simulink model "IntegratedModel"  (R2018b)
settings: Solver=ode1  StartTime=0.0  StopTime=sim.endTime_s  FixedStep=sim.timestep_s  RelTol=1e-3
undefined symbols (not defined in the file): cont, env, sim, vehicle, world
libraries: simulink x9
settings Model: Creator=ogihara  LastModifiedBy=ogihara

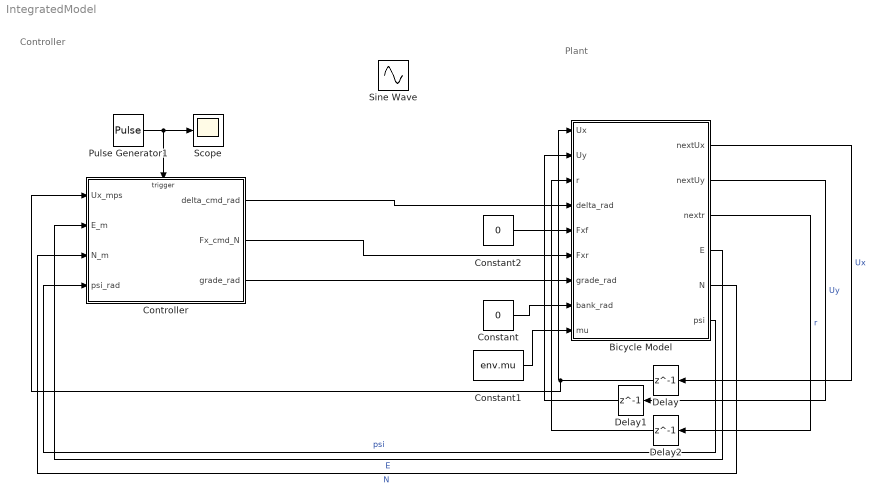
== system IntegratedModel ==
  note: Controller
  note: Plant
  Bicycle Model : Subsystem
  Constant : Constant  Value=0
  Constant1 : Constant  Value=env.mu
  Constant2 : Constant  Value=0
  Controller : Subsystem
  Delay : Delay  DelayLength=1
  Delay1 : Delay  DelayLength=1
  Delay2 : Delay  DelayLength=1
  Pulse Generator1 : DiscretePulseGenerator  PulseType=Time based  Period=cont.period  PulseWidth=10  SampleTime=sim.timestep_s
  Scope : Scope
  Sine Wave : Sin  Amplitude=20/180*pi  Frequency=1.5  SampleTime=0
  wires:
  Bicycle Model/1(nextUx) -> Delay/1  "Ux"
  Bicycle Model/2(nextUy) -> Delay1/1  "Uy"
  Bicycle Model/3(nextr) -> Delay2/1  "r"
  Bicycle Model/4(E) -> Controller/2(E_m)  "E"
  Bicycle Model/5(N) -> Controller/3(N_m)  "N"
  Bicycle Model/6(psi) -> Controller/4(psi_rad)  "psi"
  Constant1/1 -> Bicycle Model/9(mu)
  Constant/1 -> Bicycle Model/8(bank_rad)
  Delay/1 -> Bicycle Model/1(Ux), Controller/1(Ux_mps)
  Delay1/1 -> Bicycle Model/2(Uy)
  Delay2/1 -> Bicycle Model/3(r)
  Controller/3(grade_rad) -> Bicycle Model/7(grade_rad)
  Controller/2(Fx_cmd_N) -> Bicycle Model/6(Fxr)
  Controller/1(delta_cmd_rad) -> Bicycle Model/4(delta_rad)
  Constant2/1 -> Bicycle Model/5(Fxf)
  Pulse Generator1/1 -> Controller/Trigger, Scope/1

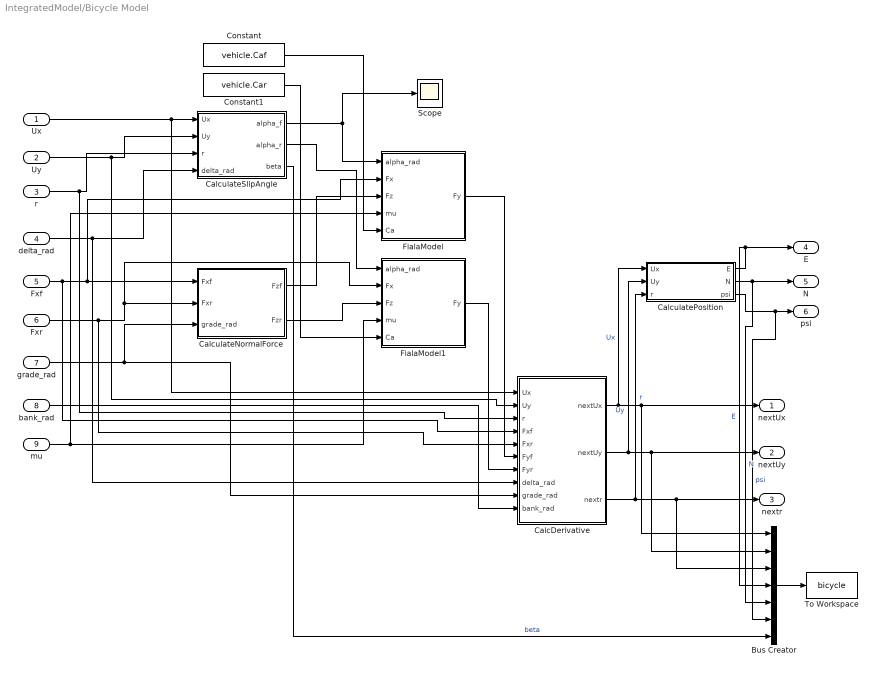
== system IntegratedModel/Bicycle Model ==
  Ux : Inport
  Uy : Inport  Port=2
  r : Inport  Port=3
  delta_rad : Inport  Port=4
  Fxf : Inport  Port=5
  Fxr : Inport  Port=6
  grade_rad : Inport  Port=7
  bank_rad : Inport  Port=8
  mu : Inport  Port=9
  Bus Creator : BusCreator  Inputs=7
  CalcDerivative : Subsystem
  CalculateNormalForce : Subsystem
  CalculatePosition : Subsystem
  CalculateSlipAngle : Subsystem
  Constant : Constant  Value=vehicle.Caf
  Constant1 : Constant  Value=vehicle.Car
  FialaModel : Subsystem
  FialaModel1 : Subsystem
  Scope : Scope
  To Workspace : ToWorkspace  VariableName=bicycle  SaveFormat=Timeseries  SampleTime=-1
  nextUx : Outport
  nextUy : Outport  Port=2
  nextr : Outport  Port=3
  E : Outport  Port=4
  N : Outport  Port=5
  psi : Outport  Port=6
  wires:
  Ux/1 -> CalcDerivative/1(Ux), CalculateSlipAngle/1(Ux)
  Uy/1 -> CalcDerivative/2(Uy), CalculateSlipAngle/2(Uy)
  r/1 -> CalcDerivative/3(r), CalculateSlipAngle/3(r)
  delta_rad/1 -> CalcDerivative/8(delta_rad), CalculateSlipAngle/4(delta_rad)
  Fxf/1 -> FialaModel/2(Fx), CalculateNormalForce/1(Fxf), CalcDerivative/4(Fxf)
  Fxr/1 -> FialaModel1/2(Fx), CalculateNormalForce/2(Fxr), CalcDerivative/5(Fxr)
  grade_rad/1 -> CalcDerivative/9(grade_rad), CalculateNormalForce/3(grade_rad)
  bank_rad/1 -> CalcDerivative/10(bank_rad)
  CalculateSlipAngle/1(alpha_f) -> FialaModel/1(alpha_rad), Scope/1
  CalculateSlipAngle/2(alpha_r) -> FialaModel1/1(alpha_rad)
  CalculateNormalForce/1(Fzf) -> FialaModel/3(Fz)
  mu/1 -> FialaModel1/4(mu), FialaModel/4(mu)
  Constant1/1 -> FialaModel1/5(Ca)
  Constant/1 -> FialaModel/5(Ca)
  CalculateNormalForce/2(Fzr) -> FialaModel1/3(Fz)
  FialaModel/1(Fy) -> CalcDerivative/6(Fyf)
  FialaModel1/1(Fy) -> CalcDerivative/7(Fyr)
  CalculatePosition/1(E) -> E/1, Bus Creator/4  "E"
  CalculatePosition/2(N) -> N/1, Bus Creator/5  "N"
  Bus Creator/1 -> To Workspace/1
  CalcDerivative/3(nextr) -> CalculatePosition/3(r), Bus Creator/3, nextr/1  "r"
  CalcDerivative/1("nextUx ") -> CalculatePosition/1(Ux), nextUx/1, Bus Creator/1  "Ux"
  CalcDerivative/2(nextUy) -> nextUy/1, Bus Creator/2, CalculatePosition/2(Uy)  "Uy"
  CalculatePosition/3(psi) -> Bus Creator/6, psi/1  "psi"
  CalculateSlipAngle/3(beta) -> Bus Creator/7  "beta"

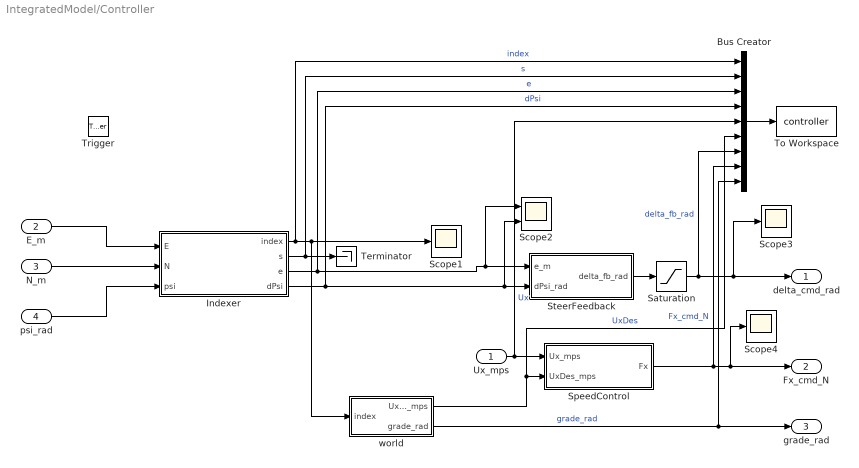
== system IntegratedModel/Controller ==
  Ux_mps : Inport
  E_m : Inport  Port=2
  N_m : Inport  Port=3
  psi_rad : Inport  Port=4
  Trigger : TriggerPort  VariantControl=Variant  PortDimensions=1
  Bus Creator : BusCreator  Inputs=9
  Indexer : Subsystem
  Saturation : Saturate  UpperLimit=vehicle.deltaMax_rad  LowerLimit=-vehicle.deltaMax_rad
  Scope1 : Scope
  Scope2 : Scope  NumInputPorts=2
  Scope3 : Scope
  Scope4 : Scope
  SpeedControl : Subsystem
  SteerFeedback : Subsystem
  Terminator : Terminator
  To Workspace : ToWorkspace  VariableName=controller  SaveFormat=Timeseries  SampleTime=-1
  world : Subsystem
  delta_cmd_rad : Outport
  Fx_cmd_N : Outport  Port=2
  grade_rad : Outport  Port=3
  wires:
  psi_rad/1 -> Indexer/3(psi)
  Indexer/1(index) -> Bus Creator/1, Scope1/1, world/1(index)  "index"
  Indexer/4(dPsi) -> Bus Creator/4, Scope2/2, SteerFeedback/2(dPsi_rad)  "dPsi"
  Indexer/3(e) -> Bus Creator/3, Scope2/1, SteerFeedback/1(e_m)  "e"
  Indexer/2(s) -> Bus Creator/2, Terminator/1  "s"
  SpeedControl/1(Fx) -> Bus Creator/8, Scope4/1, Fx_cmd_N/1  "Fx_cmd_N"
  world/2(grade_rad) -> Bus Creator/9, grade_rad/1  "grade_rad"
  Saturation/1 -> Bus Creator/7, Scope3/1, delta_cmd_rad/1  "delta_fb_rad"
  E_m/1 -> Indexer/1(E)
  N_m/1 -> Indexer/2(N)
  world/1(UxDes_mps) -> Bus Creator/6, SpeedControl/2(UxDes_mps)  "UxDes"
  Ux_mps/1 -> Bus Creator/5, SpeedControl/1(Ux_mps)  "Ux"
  SteerFeedback/1(delta_fb_rad) -> Saturation/1
  Bus Creator/1 -> To Workspace/1

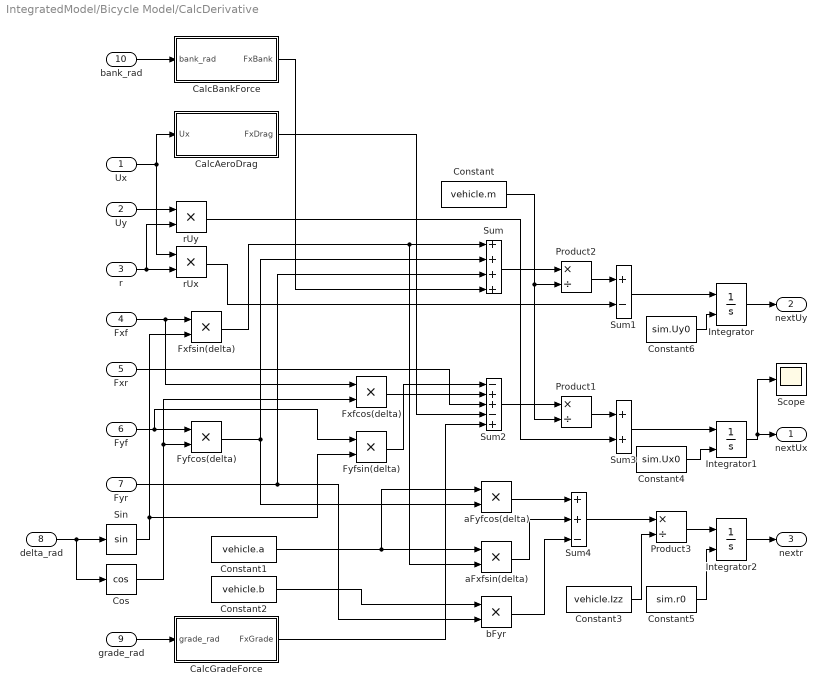
== system IntegratedModel/Bicycle Model/CalcDerivative ==
  Ux : Inport
  Uy : Inport  Port=2
  r : Inport  Port=3
  Fxf : Inport  Port=4
  Fxr : Inport  Port=5
  Fyf : Inport  Port=6
  Fyr : Inport  Port=7
  delta_rad : Inport  Port=8
  grade_rad : Inport  Port=9
  bank_rad : Inport  Port=10
  CalcAeroDrag : Subsystem
  CalcBankForce : Subsystem
  CalcGradeForce : Subsystem
  Constant : Constant  Value=vehicle.m
  Constant1 : Constant  Value=vehicle.a
  Constant2 : Constant  Value=vehicle.b
  Constant3 : Constant  Value=vehicle.Izz
  Constant4 : Constant  Value=sim.Ux0
  Constant5 : Constant  Value=sim.r0
  Constant6 : Constant  Value=sim.Uy0
  Cos : Trigonometry  Operator=cos
  Fxfcos(delta) : Product
  Fxfsin(delta) : Product
  Fyfcos(delta) : Product
  Fyfsin(delta) : Product
  Integrator : Integrator  InitialConditionSource=external
  Integrator1 : Integrator  InitialConditionSource=external
  Integrator2 : Integrator  InitialConditionSource=external  InitialCondition=sim.r0
  Product1 : Product  Inputs=*/
  Product2 : Product  Inputs=*/
  Product3 : Product  Inputs=*/
  Scope : Scope
  Sin : Trigonometry
  Sum : Sum  Inputs=++++
  Sum1 : Sum  Inputs=+-
  Sum2 : Sum  Inputs=-++-+
  Sum3 : Sum
  Sum4 : Sum  Inputs=++-
  aFxfsin(delta) : Product
  aFyfcos(delta) : Product
  bFyr : Product
  rUx : Product
  rUy : Product
  "nextUx " : Outport
  nextUy : Outport  Port=2
  nextr : Outport  Port=3
  wires:
  delta_rad/1 -> Cos/1, Sin/1
  Fyf/1 -> Fyfsin(delta)/1, Fyfcos(delta)/1
  Cos/1 -> Fxfcos(delta)/2, Fyfcos(delta)/2
  Fxf/1 -> Fxfcos(delta)/1, Fxfsin(delta)/1
  Sin/1 -> Fyfsin(delta)/2, Fxfsin(delta)/2
  Fxfsin(delta)/1 -> Sum/1, aFxfsin(delta)/2
  Fyfcos(delta)/1 -> aFyfcos(delta)/2, Sum/2
  Fyr/1 -> bFyr/2, Sum/3
  grade_rad/1 -> CalcGradeForce/1(grade_rad)
  Constant/1 -> Product1/2, Product2/2
  Sum/1 -> Product2/1
  r/1 -> rUx/2, rUy/2
  Ux/1 -> CalcAeroDrag/1(Ux), rUx/1
  Product2/1 -> Sum1/1
  Sum1/1 -> Integrator/1
  rUx/1 -> Sum1/2
  Uy/1 -> rUy/1
  bank_rad/1 -> CalcBankForce/1(bank_rad)
  CalcBankForce/1(FxBank) -> Sum/4
  Fxr/1 -> Sum2/3
  CalcAeroDrag/1(FxDrag) -> Sum2/4
  CalcGradeForce/1(FxGrade) -> Sum2/5
  Sum3/1 -> Integrator1/1
  Product1/1 -> Sum3/1
  Sum2/1 -> Product1/1
  rUy/1 -> Sum3/2
  Constant1/1 -> aFxfsin(delta)/1, aFyfcos(delta)/1
  Constant2/1 -> bFyr/1
  aFyfcos(delta)/1 -> Sum4/1
  aFxfsin(delta)/1 -> Sum4/2
  bFyr/1 -> Sum4/3
  Constant3/1 -> Product3/2
  Sum4/1 -> Product3/1
  Product3/1 -> Integrator2/1
  Integrator/1 -> nextUy/1
  Integrator1/1 -> Scope/1, "nextUx "/1
  Integrator2/1 -> nextr/1
  Constant4/1 -> Integrator1/2
  Constant5/1 -> Integrator2/2
  Constant6/1 -> Integrator/2
  Fyfsin(delta)/1 -> Sum2/1
  Fxfcos(delta)/1 -> Sum2/2

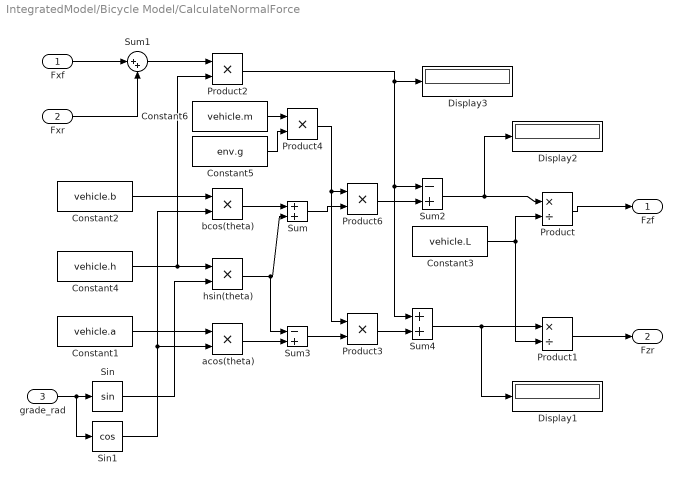
== system IntegratedModel/Bicycle Model/CalculateNormalForce ==
  Fxf : Inport
  Fxr : Inport  Port=2
  grade_rad : Inport  Port=3
  Constant1 : Constant  Value=vehicle.a
  Constant2 : Constant  Value=vehicle.b
  Constant3 : Constant  Value=vehicle.L
  Constant4 : Constant  Value=vehicle.h
  Constant5 : Constant  Value=env.g
  Constant6 : Constant  Value=vehicle.m
  Display1 : Display
  Display2 : Display
  Display3 : Display
  Product : Product  Inputs=*/
  Product1 : Product  Inputs=*/
  Product{2..4,6} (4 alike) : Product
  Sin : Trigonometry
  Sin1 : Trigonometry  Operator=cos
  Sum : Sum
  Sum1 : Sum  Inputs=|++
  Sum2 : Sum  Inputs=-+
  Sum3 : Sum  Inputs=-+
  Sum4 : Sum
  acos(theta) : Product
  bcos(theta) : Product
  hsin(theta) : Product
  Fzf : Outport
  Fzr : Outport  Port=2
  wires:
  grade_rad/1 -> Sin1/1, Sin/1
  Constant2/1 -> bcos(theta)/1
  Sin1/1 -> bcos(theta)/2, acos(theta)/2
  Constant1/1 -> acos(theta)/1
  Sin/1 -> hsin(theta)/2
  bcos(theta)/1 -> Sum/1
  hsin(theta)/1 -> Sum3/1, Sum/2
  Sum/1 -> Product6/2
  Fxf/1 -> Sum1/1
  Fxr/1 -> Sum1/2
  Constant4/1 -> Product2/2, hsin(theta)/1
  Sum1/1 -> Product2/1
  Product6/1 -> Sum2/2
  Product2/1 -> Display3/1, Sum4/1, Sum2/1
  Sum2/1 -> Display2/1, Product/1
  Product/1 -> Fzf/1
  acos(theta)/1 -> Sum3/2
  Sum4/1 -> Display1/1, Product1/1
  Product3/1 -> Sum4/2
  Sum3/1 -> Product3/2
  Product1/1 -> Fzr/1
  Constant6/1 -> Product4/1
  Constant5/1 -> Product4/2
  Product4/1 -> Product3/1, Product6/1
  Constant3/1 -> Product1/2, Product/2

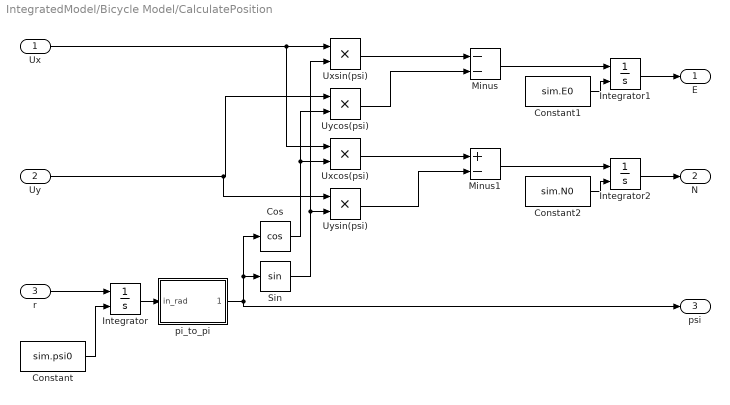
== system IntegratedModel/Bicycle Model/CalculatePosition ==
  Ux : Inport
  Uy : Inport  Port=2
  r : Inport  Port=3
  Constant : Constant  Value=sim.psi0
  Constant1 : Constant  Value=sim.E0
  Constant2 : Constant  Value=sim.N0
  Cos : Trigonometry  Operator=cos
  Integrator : Integrator  InitialConditionSource=external
  Integrator1 : Integrator  InitialConditionSource=external
  Integrator2 : Integrator  InitialConditionSource=external
  Minus : Sum  Inputs=--
  Minus1 : Sum  Inputs=+-
  Sin : Trigonometry
  Uxcos(psi) : Product
  Uxsin(psi) : Product
  Uycos(psi) : Product
  Uysin(psi) : Product
  pi_to_pi : Subsystem
  E : Outport
  N : Outport  Port=2
  psi : Outport  Port=3
  wires:
  r/1 -> Integrator/1
  Constant/1 -> Integrator/2
  Integrator/1 -> pi_to_pi/1(in_rad)
  Integrator1/1 -> E/1
  Constant1/1 -> Integrator1/2
  Ux/1 -> Uxcos(psi)/1, Uxsin(psi)/1
  Sin/1 -> Uysin(psi)/2, Uxsin(psi)/2
  Uy/1 -> Uysin(psi)/1, Uycos(psi)/1
  Cos/1 -> Uxcos(psi)/2, Uycos(psi)/2
  Uxsin(psi)/1 -> Minus/1
  Uycos(psi)/1 -> Minus/2
  Minus/1 -> Integrator1/1
  Uxcos(psi)/1 -> Minus1/1
  Uysin(psi)/1 -> Minus1/2
  Minus1/1 -> Integrator2/1
  Constant2/1 -> Integrator2/2
  Integrator2/1 -> N/1
  pi_to_pi/1(out_rad) -> Sin/1, Cos/1, psi/1

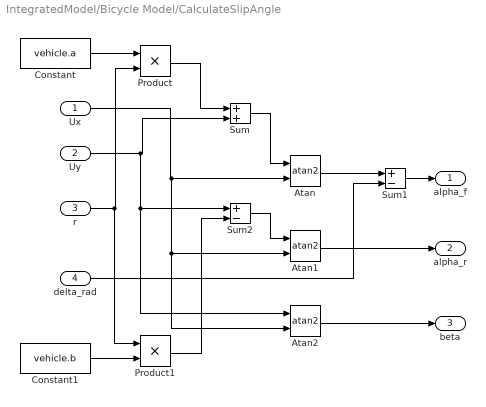
== system IntegratedModel/Bicycle Model/CalculateSlipAngle ==
  Ux : Inport
  Uy : Inport  Port=2
  r : Inport  Port=3
  delta_rad : Inport  Port=4
  Atan : Trigonometry  Operator=atan2
  Atan1 : Trigonometry  Operator=atan2
  Atan2 : Trigonometry  Operator=atan2
  Constant : Constant  Value=vehicle.a
  Constant1 : Constant  Value=vehicle.b
  Product : Product
  Product1 : Product
  Sum : Sum
  Sum1 : Sum  Inputs=+-
  Sum2 : Sum  Inputs=+-
  alpha_f : Outport
  alpha_r : Outport  Port=2
  beta : Outport  Port=3
  wires:
  Constant/1 -> Product/1
  r/1 -> Product1/1, Product/2
  Constant1/1 -> Product1/2
  Ux/1 -> Atan2/2, Atan1/2, Atan/2
  Uy/1 -> Atan2/1, Sum2/1, Sum/2
  Product/1 -> Sum/1
  Sum/1 -> Atan/1
  delta_rad/1 -> Sum1/2
  Atan/1 -> Sum1/1
  Sum1/1 -> alpha_f/1
  Product1/1 -> Sum2/2
  Sum2/1 -> Atan1/1
  Atan1/1 -> alpha_r/1
  Atan2/1 -> beta/1

== system IntegratedModel/Bicycle Model/FialaModel ==
  alpha_rad : Inport
  Fx : Inport  Port=2
  Fz : Inport  Port=3
  mu : Inport  Port=4
  Ca : Inport  Port=5
  Bus Creator : BusCreator  Inputs=7
  Switch : Switch  Criteria=u2 > Threshold
  To Workspace : ToWorkspace  VariableName=frontTire  SaveFormat=Timeseries  SampleTime=-1
  isSaturated : Subsystem
  not saturated : Subsystem
  saturated : Subsystem
  Fy : Outport
  wires:
  Switch/1 -> Bus Creator/7, Fy/1  "Fy"
  alpha_rad/1 -> Bus Creator/1, not saturated/1(alpha), isSaturated/1(alpha), saturated/4(alpha)  "alpha"
  Fx/1 -> Bus Creator/2, isSaturated/2(Fx)  "Fx"
  Fz/1 -> Bus Creator/3, not saturated/2(Fz), saturated/3(Fz), isSaturated/3(Fz)  "Fz"
  mu/1 -> saturated/1(mu), not saturated/3(mu), Bus Creator/4, isSaturated/4(mu)  "mu"
  Ca/1 -> not saturated/4(Ca), Bus Creator/5, isSaturated/5(Ca)  "Ca"
  isSaturated/1(saturatedFlag) -> Bus Creator/6, Switch/2  "isSaturated"
  saturated/1(Fy) -> Switch/1
  not saturated/1(Fy) -> Switch/3
  isSaturated/2(zeta) -> saturated/2(zeta), not saturated/5(zeta)
  Bus Creator/1 -> To Workspace/1

== system IntegratedModel/Bicycle Model/FialaModel1 ==
  alpha_rad : Inport
  Fx : Inport  Port=2
  Fz : Inport  Port=3
  mu : Inport  Port=4
  Ca : Inport  Port=5
  Bus Creator : BusCreator  Inputs=7
  Switch : Switch  Criteria=u2 > Threshold
  To Workspace : ToWorkspace  VariableName=rearTire  SaveFormat=Timeseries  SampleTime=-1
  isSaturated : Subsystem
  not saturated : Subsystem
  saturated : Subsystem
  Fy : Outport
  wires:
  Switch/1 -> Bus Creator/7, Fy/1  "Fy"
  alpha_rad/1 -> Bus Creator/1, not saturated/1(alpha), isSaturated/1(alpha), saturated/4(alpha)  "alpha"
  Fx/1 -> Bus Creator/2, isSaturated/2(Fx)  "Fx"
  Fz/1 -> Bus Creator/3, not saturated/2(Fz), saturated/3(Fz), isSaturated/3(Fz)  "Fz"
  mu/1 -> saturated/1(mu), not saturated/3(mu), Bus Creator/4, isSaturated/4(mu)  "mu"
  Ca/1 -> not saturated/4(Ca), Bus Creator/5, isSaturated/5(Ca)  "Ca"
  isSaturated/1(saturatedFlag) -> Bus Creator/6, Switch/2  "isSaturated"
  saturated/1(Fy) -> Switch/1
  not saturated/1(Fy) -> Switch/3
  isSaturated/2(zeta) -> saturated/2(zeta), not saturated/5(zeta)
  Bus Creator/1 -> To Workspace/1

== system IntegratedModel/Controller/Indexer ==
  E : Inport
  N : Inport  Port=2
  psi : Inport  Port=3
  CalcLocalCoordinate : Subsystem
  Delay1 : Delay  DelayLength=1
  FindNearestIndex : Subsystem
  IC1 : InitialCondition
  index : Outport
  s : Outport  Port=2
  e : Outport  Port=3
  dPsi : Outport  Port=4
  wires:
  IC1/1 -> FindNearestIndex/1(currentIndex)
  CalcLocalCoordinate/3(dpsi) -> dPsi/1  "dPsi"
  FindNearestIndex/1(nearestIndex) -> index/1, CalcLocalCoordinate/1(currentIdx), Delay1/1  "index"
  psi/1 -> CalcLocalCoordinate/4(psi)  "psi"
  E/1 -> CalcLocalCoordinate/2(E), FindNearestIndex/2(E)  "E"
  Delay1/1 -> IC1/1
  CalcLocalCoordinate/1(s) -> s/1  "s"
  N/1 -> CalcLocalCoordinate/3(N), FindNearestIndex/3(N)  "N"
  CalcLocalCoordinate/2(e) -> e/1  "e"

== system IntegratedModel/Controller/SpeedControl ==
  Ux_mps : Inport
  UxDes_mps : Inport  Port=2
  Gain : Gain  Gain=cont.accel_gain
  SpeedFeedback : Subsystem
  Fx : Outport
  wires:
  Ux_mps/1 -> SpeedFeedback/1(Ux_mps)
  UxDes_mps/1 -> SpeedFeedback/2(UxDes_mps)
  SpeedFeedback/1(LonCmd (-1,1)) -> Gain/1
  Gain/1 -> Fx/1  "Fx"

== system IntegratedModel/Controller/SteerFeedback ==
  e_m : Inport
  dPsi_rad : Inport  Port=2
  Gain : Gain  Gain=cont.x_la
  Gain1 : Gain  Gain=cont.k_fb
  Plus : Sum
  delta_fb_rad : Outport
  wires:
  dPsi_rad/1 -> Gain/1
  e_m/1 -> Plus/1
  Gain/1 -> Plus/2
  Plus/1 -> Gain1/1
  Gain1/1 -> delta_fb_rad/1

== system IntegratedModel/Controller/world ==
  index : Inport
  world.UxDes_mps : Lookup_n-D  NumberOfTableDimensions=1  BreakpointsForDimension1=world.index  Table=world.UxDes_mps  InternalRulePriority=Speed  RndMeth=Simplest  InputSameDT=on
  world.grade_rad : Lookup_n-D  NumberOfTableDimensions=1  BreakpointsForDimension1=world.index  Table=world.grade_rad  InternalRulePriority=Speed  RndMeth=Simplest  InputSameDT=on
  UxDes_mps : Outport
  grade_rad : Outport  Port=2
  wires:
  index/1 -> world.UxDes_mps/1, world.grade_rad/1
  world.grade_rad/1 -> grade_rad/1  "grade"
  world.UxDes_mps/1 -> UxDes_mps/1  "UxDes"

== system IntegratedModel/Bicycle Model/CalcDerivative/CalcAeroDrag ==
  Ux : Inport
  Constant : Constant  Value=vehicle.Cd0
  Gain : Gain  Gain=vehicle.Cd1
  Gain1 : Gain  Gain=vehicle.Cd2
  Product : Product
  Product1 : Product
  Sign : Signum
  Square : Math  Operator=square  SaturateOnIntegerOverflow=on
  Sum : Sum  Inputs=3
  FxDrag : Outport
  wires:
  Sum/1 -> FxDrag/1
  Gain1/1 -> Product1/2
  Gain/1 -> Sum/2
  Square/1 -> Gain1/1
  Ux/1 -> Gain/1, Square/1, Sign/1
  Product/1 -> Sum/1
  Sign/1 -> Product1/1, Product/2
  Constant/1 -> Product/1
  Product1/1 -> Sum/3

== system IntegratedModel/Bicycle Model/CalcDerivative/CalcBankForce ==
  bank_rad : Inport
  Constant : Constant  Value=vehicle.m
  Constant1 : Constant  Value=env.g
  Product : Product  Inputs=3
  Sin : Trigonometry
  FxBank : Outport
  wires:
  bank_rad/1 -> Sin/1
  Sin/1 -> Product/1
  Constant/1 -> Product/2
  Constant1/1 -> Product/3
  Product/1 -> FxBank/1

== system IntegratedModel/Bicycle Model/CalcDerivative/CalcGradeForce ==
  grade_rad : Inport
  Constant : Constant  Value=vehicle.m
  Constant1 : Constant  Value=env.g
  Product : Product  Inputs=3
  Sin : Trigonometry
  FxGrade : Outport
  wires:
  grade_rad/1 -> Sin/1
  Sin/1 -> Product/1
  Constant/1 -> Product/2
  Constant1/1 -> Product/3
  Product/1 -> FxGrade/1

== system IntegratedModel/Bicycle Model/CalculatePosition/pi_to_pi ==
  in_rad : Inport
  Compare To Constant : simulink/Logic and Bit Operations/Compare To Constant  relop=<=  const=-pi  OutDataTypeStr=boolean
  Compare To Constant1 : simulink/Logic and Bit Operations/Compare To Constant  relop=>  const=pi  OutDataTypeStr=boolean
  Constant : Constant  Value=2*pi
  Minus : Sum  Inputs=+-
  Plus : Sum
  Switch : Switch  Criteria=u2 > Threshold
  Switch1 : Switch  Criteria=u2 > Threshold
  out_rad : Outport
  wires:
  Constant/1 -> Minus/2, Plus/2
  in_rad/1 -> Switch/3, Compare To Constant/1, Minus/1, Plus/1
  Compare To Constant1/1 -> Switch1/2
  Compare To Constant/1 -> Switch/2
  Plus/1 -> Switch/1
  Switch/1 -> Switch1/3, Compare To Constant1/1
  Minus/1 -> Switch1/1
  Switch1/1 -> out_rad/1

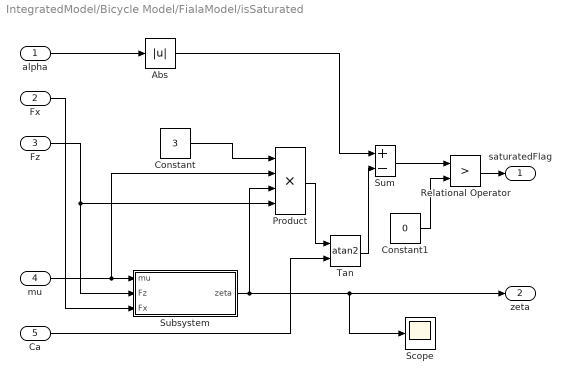
== system IntegratedModel/Bicycle Model/FialaModel/isSaturated ==
  alpha : Inport
  Fx : Inport  Port=2
  Fz : Inport  Port=3
  mu : Inport  Port=4
  Ca : Inport  Port=5
  Abs : Abs
  Constant : Constant  Value=3
  Constant1 : Constant  Value=0
  Product : Product  Inputs=4
  Relational Operator : RelationalOperator  Operator=>  OutDataTypeStr=boolean  RndMeth=Simplest
  Scope : Scope
  Subsystem : Subsystem
  Sum : Sum  Inputs=+-
  Tan : Trigonometry  Operator=atan2
  saturatedFlag : Outport
  zeta : Outport  Port=2
  wires:
  Subsystem/1(zeta) -> Scope/1, zeta/1, Product/3
  Product/1 -> Tan/1
  Tan/1 -> Sum/2
  Fx/1 -> Subsystem/3(Fx)
  Fz/1 -> Subsystem/2(Fz), Product/4
  Constant/1 -> Product/1
  mu/1 -> Product/2, Subsystem/1(mu)
  Ca/1 -> Tan/2
  Abs/1 -> Sum/1
  alpha/1 -> Abs/1
  Sum/1 -> Relational Operator/1
  Constant1/1 -> Relational Operator/2
  Relational Operator/1 -> saturatedFlag/1

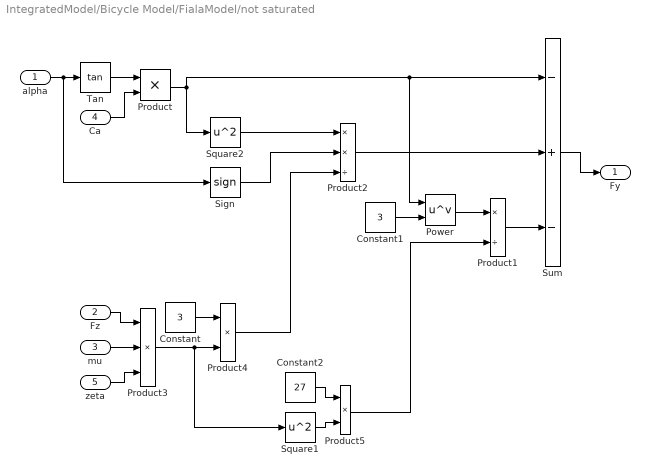
== system IntegratedModel/Bicycle Model/FialaModel/not saturated ==
  alpha : Inport
  Fz : Inport  Port=2
  mu : Inport  Port=3
  Ca : Inport  Port=4
  zeta : Inport  Port=5
  Constant : Constant  Value=3
  Constant1 : Constant  Value=3
  Constant2 : Constant  Value=27
  Power : Math  Operator=pow  SaturateOnIntegerOverflow=on
  Product : Product
  Product1 : Product  Inputs=*/
  Product2 : Product  Inputs=**/
  Product3 : Product  Inputs=***
  Product4 : Product
  Product5 : Product
  Sign : Signum
  Square1 : Math  Operator=square  SaturateOnIntegerOverflow=on
  Square2 : Math  Operator=square  SaturateOnIntegerOverflow=on
  Sum : Sum  Inputs=-+-
  Tan : Trigonometry  Operator=tan
  Fy : Outport
  wires:
  Sum/1 -> Fy/1
  alpha/1 -> Sign/1, Tan/1
  Tan/1 -> Product/1
  Ca/1 -> Product/2
  Product/1 -> Square2/1, Power/1, Sum/1
  Square2/1 -> Product2/1
  Product2/1 -> Sum/2
  Fz/1 -> Product3/1
  mu/1 -> Product3/2
  zeta/1 -> Product3/3
  Product3/1 -> Square1/1, Product4/2
  Constant/1 -> Product4/1
  Product4/1 -> Product2/3
  Sign/1 -> Product2/2
  Constant2/1 -> Product5/1
  Square1/1 -> Product5/2
  Constant1/1 -> Power/2
  Power/1 -> Product1/1
  Product5/1 -> Product1/2
  Product1/1 -> Sum/3

== system IntegratedModel/Bicycle Model/FialaModel/saturated ==
  mu : Inport
  zeta : Inport  Port=2
  Fz : Inport  Port=3
  alpha : Inport  Port=4
  Gain : Gain  Gain=-1
  Product : Product  Inputs=4
  Sign : Signum
  Fy : Outport
  wires:
  alpha/1 -> Sign/1
  Product/1 -> Gain/1
  Gain/1 -> Fy/1
  mu/1 -> Product/1
  zeta/1 -> Product/2
  Fz/1 -> Product/3
  Sign/1 -> Product/4

== system IntegratedModel/Bicycle Model/FialaModel1/isSaturated ==
  alpha : Inport
  Fx : Inport  Port=2
  Fz : Inport  Port=3
  mu : Inport  Port=4
  Ca : Inport  Port=5
  Abs : Abs
  Constant : Constant  Value=3
  Constant1 : Constant  Value=0
  Product : Product  Inputs=4
  Relational Operator : RelationalOperator  Operator=>  OutDataTypeStr=boolean  RndMeth=Simplest
  Scope : Scope
  Subsystem : Subsystem
  Sum : Sum  Inputs=+-
  Tan : Trigonometry  Operator=atan2
  saturatedFlag : Outport
  zeta : Outport  Port=2
  wires:
  Subsystem/1(zeta) -> Scope/1, zeta/1, Product/3
  Product/1 -> Tan/1
  Tan/1 -> Sum/2
  Fx/1 -> Subsystem/3(Fx)
  Fz/1 -> Subsystem/2(Fz), Product/4
  Constant/1 -> Product/1
  mu/1 -> Product/2, Subsystem/1(mu)
  Ca/1 -> Tan/2
  Abs/1 -> Sum/1
  alpha/1 -> Abs/1
  Sum/1 -> Relational Operator/1
  Constant1/1 -> Relational Operator/2
  Relational Operator/1 -> saturatedFlag/1

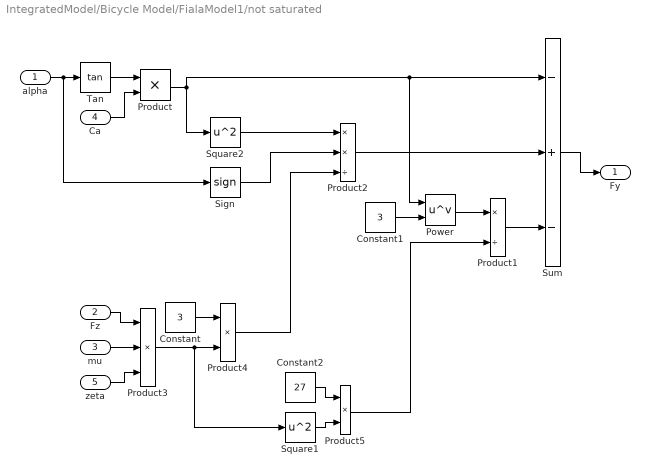
== system IntegratedModel/Bicycle Model/FialaModel1/not saturated ==
  alpha : Inport
  Fz : Inport  Port=2
  mu : Inport  Port=3
  Ca : Inport  Port=4
  zeta : Inport  Port=5
  Constant : Constant  Value=3
  Constant1 : Constant  Value=3
  Constant2 : Constant  Value=27
  Power : Math  Operator=pow  SaturateOnIntegerOverflow=on
  Product : Product
  Product1 : Product  Inputs=*/
  Product2 : Product  Inputs=**/
  Product3 : Product  Inputs=***
  Product4 : Product
  Product5 : Product
  Sign : Signum
  Square1 : Math  Operator=square  SaturateOnIntegerOverflow=on
  Square2 : Math  Operator=square  SaturateOnIntegerOverflow=on
  Sum : Sum  Inputs=-+-
  Tan : Trigonometry  Operator=tan
  Fy : Outport
  wires:
  Sum/1 -> Fy/1
  alpha/1 -> Sign/1, Tan/1
  Tan/1 -> Product/1
  Ca/1 -> Product/2
  Product/1 -> Square2/1, Power/1, Sum/1
  Square2/1 -> Product2/1
  Product2/1 -> Sum/2
  Fz/1 -> Product3/1
  mu/1 -> Product3/2
  zeta/1 -> Product3/3
  Product3/1 -> Square1/1, Product4/2
  Constant/1 -> Product4/1
  Product4/1 -> Product2/3
  Sign/1 -> Product2/2
  Constant2/1 -> Product5/1
  Square1/1 -> Product5/2
  Constant1/1 -> Power/2
  Power/1 -> Product1/1
  Product5/1 -> Product1/2
  Product1/1 -> Sum/3

== system IntegratedModel/Bicycle Model/FialaModel1/saturated ==
  mu : Inport
  zeta : Inport  Port=2
  Fz : Inport  Port=3
  alpha : Inport  Port=4
  Gain : Gain  Gain=-1
  Product : Product  Inputs=4
  Sign : Signum
  Fy : Outport
  wires:
  alpha/1 -> Sign/1
  Product/1 -> Gain/1
  Gain/1 -> Fy/1
  mu/1 -> Product/1
  zeta/1 -> Product/2
  Fz/1 -> Product/3
  Sign/1 -> Product/4

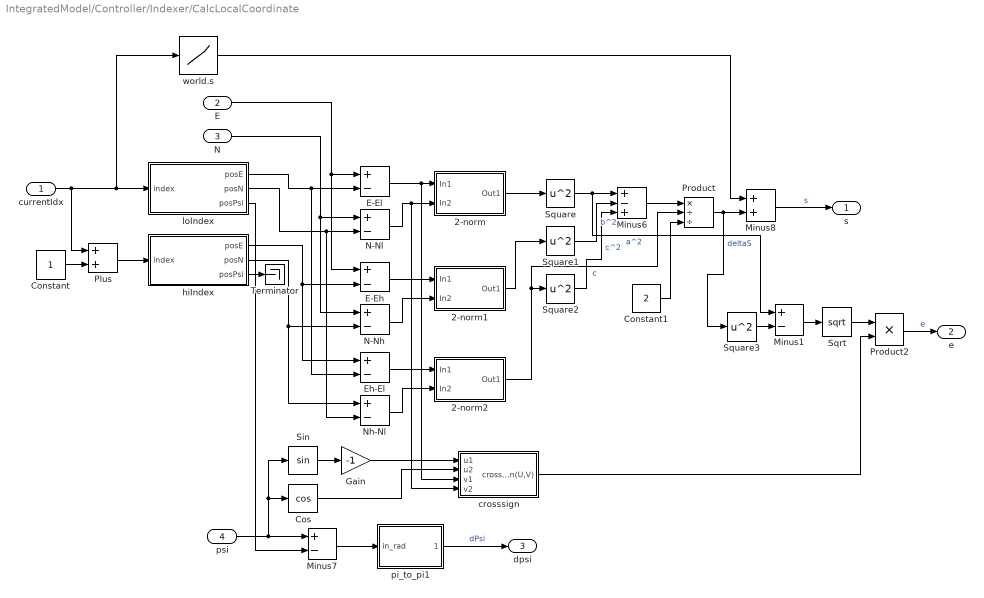
== system IntegratedModel/Controller/Indexer/CalcLocalCoordinate ==
  currentIdx : Inport
  E : Inport  Port=2
  N : Inport  Port=3
  psi : Inport  Port=4
  2-norm : Subsystem
  2-norm1 : Subsystem
  2-norm2 : Subsystem
  Constant : Constant
  Constant1 : Constant  Value=2
  Cos : Trigonometry  Operator=cos
  E-Eh : Sum  Inputs=+-
  E-El : Sum  Inputs=+-
  Eh-El : Sum  Inputs=+-
  Gain : Gain  Gain=-1
  Minus1 : Sum  Inputs=+-
  Minus6 : Sum  Inputs=+-+
  Minus7 : Sum  Inputs=+-
  Minus8 : Sum
  N-Nh : Sum  Inputs=+-
  N-Nl : Sum  Inputs=+-
  Nh-Nl : Sum  Inputs=+-
  Plus : Sum
  Product : Product  Inputs=*//
  Product2 : Product
  Sin : Trigonometry
  Sqrt : Sqrt  SaturateOnIntegerOverflow=on
  Square{,1..3} (4 alike) : Math  Operator=square  SaturateOnIntegerOverflow=on
  Terminator : Terminator
  crosssign : Subsystem
  hiIndex : Subsystem
  loIndex : Subsystem
  pi_to_pi1 : Subsystem
  world.s : Lookup_n-D  NumberOfTableDimensions=1  BreakpointsForDimension1=world.index  Table=world.s_m  InternalRulePriority=Speed  RndMeth=Simplest  InputSameDT=on
  s : Outport
  e : Outport  Port=2
  dpsi : Outport  Port=3
  wires:
  currentIdx/1 -> Plus/1, world.s/1, loIndex/1(index)
  Constant/1 -> Plus/2
  Plus/1 -> hiIndex/1(index)
  hiIndex/3(posPsi) -> Terminator/1
  hiIndex/1(posE) -> Eh-El/1, E-Eh/2
  E-El/1 -> crosssign/3(v1), 2-norm/1(In1)
  N-Nl/1 -> crosssign/4(v2), 2-norm/2(In2)
  E-Eh/1 -> 2-norm1/1(In1)
  N-Nh/1 -> 2-norm1/2(In2)
  Eh-El/1 -> 2-norm2/1(In1)
  Nh-Nl/1 -> 2-norm2/2(In2)
  2-norm/1(Out1) -> Square/1
  2-norm1/1(Out1) -> Square1/1
  2-norm2/1(Out1) -> Product/2, Square2/1  "c"
  Square/1 -> Minus1/1, Minus6/1  "a^2"
  Square1/1 -> Minus6/2  "b^2"
  Square2/1 -> Minus6/3  "c^2"
  Minus6/1 -> Product/1
  Constant1/1 -> Product/3
  psi/1 -> Cos/1, Sin/1, Minus7/1
  Minus7/1 -> pi_to_pi1/1(in_rad)
  Product/1 -> Square3/1, Minus8/2  "deltaS"
  world.s/1 -> Minus8/1
  Minus8/1 -> s/1  "s"
  Sin/1 -> Gain/1
  Gain/1 -> crosssign/1(u1)
  Cos/1 -> crosssign/2(u2)
  E/1 -> E-Eh/1, E-El/1
  loIndex/1(posE) -> Eh-El/2, E-El/2
  loIndex/2(posN) -> Nh-Nl/2, N-Nl/2
  N/1 -> N-Nh/1, N-Nl/1
  hiIndex/2(posN) -> Nh-Nl/1, N-Nh/2
  loIndex/3(posPsi) -> Minus7/2
  Square3/1 -> Minus1/2
  Minus1/1 -> Sqrt/1
  Sqrt/1 -> Product2/1
  Product2/1 -> e/1  "e"
  crosssign/1(crosssign(U,V)) -> Product2/2
  pi_to_pi1/1(out_rad) -> dpsi/1  "dPsi"

== system IntegratedModel/Controller/Indexer/FindNearestIndex ==
  note: Osprey had forward & backward search.
      | This simulator has only forward search and max width is 5.
  currentIndex : Inport
  E : Inport  Port=2
  N : Inport  Port=3
  ForwardSearch : Subsystem  TreatAsAtomicUnit=on
  nearestIndex : Outport
  wires:
  currentIndex/1 -> ForwardSearch/1(CurrentIndex)
  E/1 -> ForwardSearch/2(E)
  N/1 -> ForwardSearch/3(N)
  ForwardSearch/1(loIndexF) -> nearestIndex/1

== system IntegratedModel/Controller/SpeedControl/SpeedFeedback ==
  Ux_mps : Inport
  UxDes_mps : Inport  Port=2
  Gain : Gain  Gain=cont.speed_gain
  PID Controller : simulink/Continuous/PID Controller  Controller=PID  Form=Parallel  TimeDomain=Discrete-time  SampleTime=-1  IntegratorMethod=Forward Euler  FilterMethod=Forward Euler  ControllerParametersSource=internal  P=cont.k_p_speed  I=cont.k_i_speed  D=cont.k_d_speed  UseFilter=on  N=100  TunerSelectOption=Transfer Function Based (PID Tuner App)  InitialConditionSource=internal  InitialConditionForIntegrator=0  InitialConditionForFilter=0  DifferentiatorICPrevScaledInput=0  ExternalReset=none  TrackingMode=off  Kt=1  LimitOutput=off  UpperSaturationLimit=inf  LowerSaturationLimit=-inf  LinearizeAsGain=on  AntiWindupMode=none  Kb=1  POutMin=[]  POutMax=[]  IOutMin=[]  IOutMax=[]  DOutMin=[]  DOutMax=[]  NOutMin=[]  NOutMax=[]  SumOutMin=[]  SumOutMax=[]  SaturationOutMin=[]  SaturationOutMax=[]  PParamMin=[]  PParamMax=[]  IParamMin=[]  IParamMax=[]  DParamMin=[]  DParamMax=[]  NParamMin=[]  NParamMax=[]  KbParamMin=[]  KbParamMax=[]  KtParamMin=[]  KtParamMax=[]  KbOutMin=[]  KbOutMax=[]  KtOutMin=[]  KtOutMax=[]  IntegratorOutMin=[]  IntegratorOutMax=[]  FilterOutMin=[]  FilterOutMax=[]  SumI1OutMin=[]  SumI1OutMax=[]  SumI2OutMin=[]  SumI2OutMax=[]  SumI3OutMin=[]  SumI3OutMax=[]  SumI4OutMin=[]  SumI4OutMax=[]  SumDOutMin=[]  SumDOutMax=[]  DifferentiatorOutMin=[]  DifferentiatorOutMax=[]  FilterDiffOutCoefMin=[]  FilterDiffOutCoefMax=[]  ReciprocalOutMin=[]  ReciprocalOutMax=[]  SumDenOutMin=[]  SumDenOutMax=[]  SumNumOutMin=[]  SumNumOutMax=[]  DivideOutMin=[]  DivideOutMax=[]  IntegratorContinuousStateAttributes=''  IntegratorStateMustResolveToSignalObject=off  IntegratorRTWStateStorageClass=Auto  FilterContinuousStateAttributes=''  FilterStateMustResolveToSignalObject=off  FilterRTWStateStorageClass=Auto  ParallelPVariant=InternalParameters  IdealPVariant=Disabled  IVariant=InternalParameters  DVariant=InternalParameters  IntegratorVariant=Discrete  SatVariant=Disabled  AWVariant=Passthrough  PCopyVariant=Disabled  TRVariant=Disabled  FdbkBlocksVariant=Forward  IdealPFdbkVariant=Disabled  SatFdbkVariant=Disabled  DerivativeFilterVariant=ForwardEulerFilter  NVariant=InternalParameters  NCopyVariant=Disabled  FilterICVariant=InternalICsFilter  IntegratorICVariant=InternalICs  ExternalResetVariant=Disabled  TRSumVariant=Passthrough  SumFdbkVariant=Disabled  SumVariant=Sum_PID
  Plus : Sum  Inputs=+-
  Saturation : Saturate  UpperLimit=+1  LowerLimit=-1
  Scope : Scope  NumInputPorts=2
  LonCmd (-1,1) : Outport
  wires:
  PID Controller/1 -> Gain/1
  Gain/1 -> Saturation/1
  Saturation/1 -> Scope/2, LonCmd (-1,1)/1
  Ux_mps/1 -> Plus/2
  UxDes_mps/1 -> Plus/1
  Plus/1 -> Scope/1, PID Controller/1

== system IntegratedModel/Bicycle Model/FialaModel/isSaturated/Subsystem ==
  mu : Inport
  Fz : Inport  Port=2
  Fx : Inport  Port=3
  Product : Product
  Product1 : Product  Inputs=*/
  Product2 : Product
  Sqrt : Sqrt  SaturateOnIntegerOverflow=on
  Square : Math  Operator=square  SaturateOnIntegerOverflow=on
  Square1 : Math  Operator=square  SaturateOnIntegerOverflow=on
  Square2 : Math  Operator=square  SaturateOnIntegerOverflow=on
  Sum : Sum  Inputs=+-
  zeta : Outport
  wires:
  mu/1 -> Product2/1, Square1/1
  Fz/1 -> Product2/2, Square/1
  Fx/1 -> Square2/1
  Square1/1 -> Product/1
  Square/1 -> Product/2
  Product/1 -> Sum/1
  Square2/1 -> Sum/2
  Sum/1 -> Sqrt/1
  Sqrt/1 -> Product1/1
  Product2/1 -> Product1/2
  Product1/1 -> zeta/1

== system IntegratedModel/Bicycle Model/FialaModel1/isSaturated/Subsystem ==
  mu : Inport
  Fz : Inport  Port=2
  Fx : Inport  Port=3
  Product : Product
  Product1 : Product  Inputs=*/
  Product2 : Product
  Sqrt : Sqrt  SaturateOnIntegerOverflow=on
  Square : Math  Operator=square  SaturateOnIntegerOverflow=on
  Square1 : Math  Operator=square  SaturateOnIntegerOverflow=on
  Square2 : Math  Operator=square  SaturateOnIntegerOverflow=on
  Sum : Sum  Inputs=+-
  zeta : Outport
  wires:
  mu/1 -> Product2/1, Square1/1
  Fz/1 -> Product2/2, Square/1
  Fx/1 -> Square2/1
  Square1/1 -> Product/1
  Square/1 -> Product/2
  Product/1 -> Sum/1
  Square2/1 -> Sum/2
  Sum/1 -> Sqrt/1
  Sqrt/1 -> Product1/1
  Product2/1 -> Product1/2
  Product1/1 -> zeta/1

== system IntegratedModel/Controller/Indexer/CalcLocalCoordinate/2-norm ==
  In1 : Inport
  In2 : Inport  Port=2
  Plus : Sum
  Sqrt : Sqrt  SaturateOnIntegerOverflow=on
  Square : Math  Operator=square  SaturateOnIntegerOverflow=on
  Square1 : Math  Operator=square  SaturateOnIntegerOverflow=on
  Out1 : Outport
  wires:
  In1/1 -> Square/1
  In2/1 -> Square1/1
  Square/1 -> Plus/1
  Square1/1 -> Plus/2
  Plus/1 -> Sqrt/1
  Sqrt/1 -> Out1/1

== system IntegratedModel/Controller/Indexer/CalcLocalCoordinate/2-norm1 ==
  In1 : Inport
  In2 : Inport  Port=2
  Plus : Sum
  Sqrt : Sqrt  SaturateOnIntegerOverflow=on
  Square : Math  Operator=square  SaturateOnIntegerOverflow=on
  Square1 : Math  Operator=square  SaturateOnIntegerOverflow=on
  Out1 : Outport
  wires:
  In1/1 -> Square/1
  In2/1 -> Square1/1
  Square/1 -> Plus/1
  Square1/1 -> Plus/2
  Plus/1 -> Sqrt/1
  Sqrt/1 -> Out1/1

== system IntegratedModel/Controller/Indexer/CalcLocalCoordinate/2-norm2 ==
  In1 : Inport
  In2 : Inport  Port=2
  Plus : Sum
  Sqrt : Sqrt  SaturateOnIntegerOverflow=on
  Square : Math  Operator=square  SaturateOnIntegerOverflow=on
  Square1 : Math  Operator=square  SaturateOnIntegerOverflow=on
  Out1 : Outport
  wires:
  In1/1 -> Square/1
  In2/1 -> Square1/1
  Square/1 -> Plus/1
  Square1/1 -> Plus/2
  Plus/1 -> Sqrt/1
  Sqrt/1 -> Out1/1

== system IntegratedModel/Controller/Indexer/CalcLocalCoordinate/crosssign ==
  note: U = (u1,u2), V=(v1,v2)
      | if V is equal to or more left than U, then crosssign is +1
      | else, crosssign is -1.
      |
      | cross sign is sgn(cross(a,b))
  u1 : Inport
  u2 : Inport  Port=2
  v1 : Inport  Port=3
  v2 : Inport  Port=4
  Minus : Sum  Inputs=+-
  Product : Product
  Product1 : Product
  Sign : Signum
  crosssign(U,V) : Outport
  wires:
  Minus/1 -> Sign/1
  Sign/1 -> crosssign(U,V)/1
  u1/1 -> Product/1
  v2/1 -> Product/2
  u2/1 -> Product1/1
  v1/1 -> Product1/2
  Product/1 -> Minus/1
  Product1/1 -> Minus/2

== system IntegratedModel/Controller/Indexer/CalcLocalCoordinate/hiIndex ==
  index : Inport
  world.posE_m : Lookup_n-D  NumberOfTableDimensions=1  BreakpointsForDimension1=world.index  Table=world.posE_m  InternalRulePriority=Speed  RndMeth=Simplest  InputSameDT=on
  world.posN_m : Lookup_n-D  NumberOfTableDimensions=1  BreakpointsForDimension1=world.index  Table=world.posN_m  InternalRulePriority=Speed  RndMeth=Simplest  InputSameDT=on
  world.psi_rad : Lookup_n-D  NumberOfTableDimensions=1  BreakpointsForDimension1=world.index  Table=world.psi_rad  InternalRulePriority=Speed  RndMeth=Simplest  InputSameDT=on
  posE : Outport
  posN : Outport  Port=2
  posPsi : Outport  Port=3
  wires:
  world.psi_rad/1 -> posPsi/1
  index/1 -> world.psi_rad/1, world.posN_m/1, world.posE_m/1
  world.posE_m/1 -> posE/1
  world.posN_m/1 -> posN/1

== system IntegratedModel/Controller/Indexer/CalcLocalCoordinate/loIndex ==
  index : Inport
  world.posE_m : Lookup_n-D  NumberOfTableDimensions=1  BreakpointsForDimension1=world.index  Table=world.posE_m  InternalRulePriority=Speed  RndMeth=Simplest  InputSameDT=on
  world.posN_m : Lookup_n-D  NumberOfTableDimensions=1  BreakpointsForDimension1=world.index  Table=world.posN_m  InternalRulePriority=Speed  RndMeth=Simplest  InputSameDT=on
  world.psi_rad : Lookup_n-D  NumberOfTableDimensions=1  BreakpointsForDimension1=world.index  Table=world.psi_rad  InternalRulePriority=Speed  RndMeth=Simplest  InputSameDT=on
  posE : Outport
  posN : Outport  Port=2
  posPsi : Outport  Port=3
  wires:
  world.psi_rad/1 -> posPsi/1
  index/1 -> world.psi_rad/1, world.posN_m/1, world.posE_m/1
  world.posE_m/1 -> posE/1
  world.posN_m/1 -> posN/1

== system IntegratedModel/Controller/Indexer/CalcLocalCoordinate/pi_to_pi1 ==
  in_rad : Inport
  Compare To Constant : simulink/Logic and Bit Operations/Compare To Constant  relop=<=  const=-pi  OutDataTypeStr=boolean
  Compare To Constant1 : simulink/Logic and Bit Operations/Compare To Constant  relop=>  const=pi  OutDataTypeStr=boolean
  Constant : Constant  Value=2*pi
  Minus : Sum  Inputs=+-
  Plus : Sum
  Switch : Switch  Criteria=u2 > Threshold
  Switch1 : Switch  Criteria=u2 > Threshold
  out_rad : Outport
  wires:
  Constant/1 -> Minus/2, Plus/2
  in_rad/1 -> Switch/3, Compare To Constant/1, Minus/1, Plus/1
  Compare To Constant1/1 -> Switch1/2
  Compare To Constant/1 -> Switch/2
  Plus/1 -> Switch/1
  Switch/1 -> Switch1/3, Compare To Constant1/1
  Minus/1 -> Switch1/1
  Switch1/1 -> out_rad/1

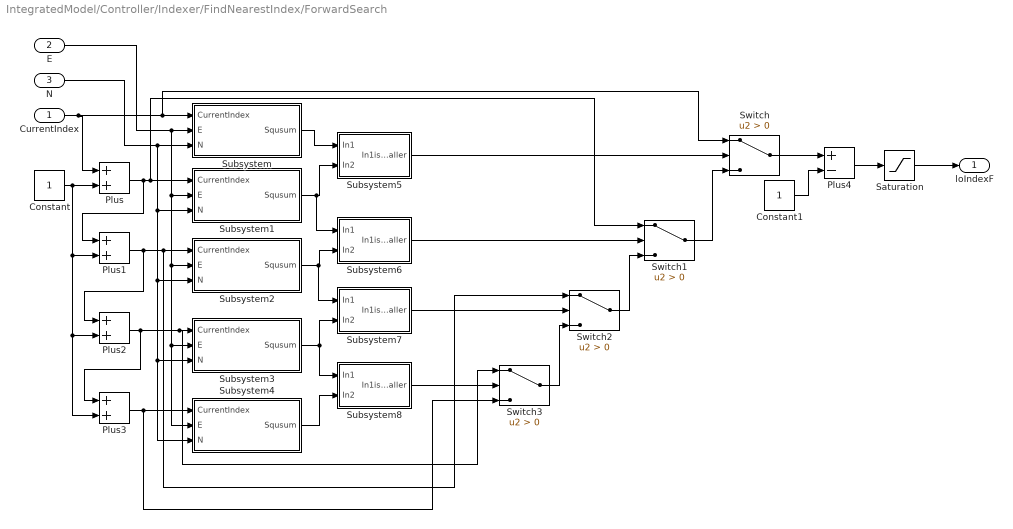
== system IntegratedModel/Controller/Indexer/FindNearestIndex/ForwardSearch ==
  CurrentIndex : Inport
  E : Inport  Port=2
  N : Inport  Port=3
  Constant : Constant
  Constant1 : Constant
  Plus{,1..3} (4 alike) : Sum
  Plus4 : Sum  Inputs=+-
  Saturation : Saturate  UpperLimit=world.maxIndex  LowerLimit=1
  Subsystem : Subsystem
  Subsystem1 : Subsystem
  Subsystem2 : Subsystem
  Subsystem3 : Subsystem
  Subsystem4 : Subsystem
  Subsystem5 : Subsystem
  Subsystem6 : Subsystem
  Subsystem7 : Subsystem
  Subsystem8 : Subsystem
  Switch{,1..3} (4 alike) : Switch  Criteria=u2 > Threshold
  loIndexF : Outport
  wires:
  Constant/1 -> Plus2/2, Plus3/2, Plus1/2, Plus/2
  CurrentIndex/1 -> Plus/1, Switch/1, Subsystem/1(CurrentIndex)
  Plus/1 -> Subsystem1/1(CurrentIndex), Switch1/1, Plus1/1
  E/1 -> Subsystem1/2(E), Subsystem2/2(E), Subsystem4/2(E), Subsystem3/2(E), Subsystem/2(E)
  N/1 -> Subsystem1/3(N), Subsystem2/3(N), Subsystem4/3(N), Subsystem3/3(N), Subsystem/3(N)
  Plus1/1 -> Plus2/1, Subsystem2/1(CurrentIndex), Switch2/1
  Plus2/1 -> Switch3/1, Subsystem3/1(CurrentIndex), Plus3/1
  Subsystem/1(Squsum) -> Subsystem5/1(In1)
  Subsystem1/1(Squsum) -> Subsystem6/1(In1), Subsystem5/2(In2)
  Subsystem2/1(Squsum) -> Subsystem7/1(In1), Subsystem6/2(In2)
  Subsystem3/1(Squsum) -> Subsystem8/1(In1), Subsystem7/2(In2)
  Subsystem4/1(Squsum) -> Subsystem8/2(In2)
  Subsystem5/1(In1isSmaller) -> Switch/2
  Subsystem6/1(In1isSmaller) -> Switch1/2
  Subsystem7/1(In1isSmaller) -> Switch2/2
  Subsystem8/1(In1isSmaller) -> Switch3/2
  Switch/1 -> Plus4/1
  Switch1/1 -> Switch/3
  Switch2/1 -> Switch1/3
  Switch3/1 -> Switch2/3
  Plus3/1 -> Subsystem4/1(CurrentIndex), Switch3/3
  Plus4/1 -> Saturation/1
  Saturation/1 -> loIndexF/1
  Constant1/1 -> Plus4/2

== system IntegratedModel/Controller/Indexer/FindNearestIndex/ForwardSearch/Subsystem ==
  CurrentIndex : Inport
  E : Inport  Port=2
  N : Inport  Port=3
  Saturation : Saturate  UpperLimit=world.maxIndex  LowerLimit=1
  squaresum : Subsystem
  world : Subsystem
  Squsum : Outport
  wires:
  squaresum/1(squsum) -> Squsum/1
  CurrentIndex/1 -> Saturation/1
  N/1 -> squaresum/4(N2)
  world/1(posE) -> squaresum/1(E1)
  E/1 -> squaresum/3(E2)
  world/2(posN) -> squaresum/2(N1)
  Saturation/1 -> world/1(index)

== system IntegratedModel/Controller/Indexer/FindNearestIndex/ForwardSearch/Subsystem1 ==
  CurrentIndex : Inport
  E : Inport  Port=2
  N : Inport  Port=3
  Saturation : Saturate  UpperLimit=world.maxIndex  LowerLimit=1
  squaresum : Subsystem
  world : Subsystem
  Squsum : Outport
  wires:
  squaresum/1(squsum) -> Squsum/1
  CurrentIndex/1 -> Saturation/1
  N/1 -> squaresum/4(N2)
  world/1(posE) -> squaresum/1(E1)
  E/1 -> squaresum/3(E2)
  world/2(posN) -> squaresum/2(N1)
  Saturation/1 -> world/1(index)

== system IntegratedModel/Controller/Indexer/FindNearestIndex/ForwardSearch/Subsystem2 ==
  CurrentIndex : Inport
  E : Inport  Port=2
  N : Inport  Port=3
  Saturation : Saturate  UpperLimit=world.maxIndex  LowerLimit=1
  squaresum : Subsystem
  world : Subsystem
  Squsum : Outport
  wires:
  squaresum/1(squsum) -> Squsum/1
  CurrentIndex/1 -> Saturation/1
  N/1 -> squaresum/4(N2)
  world/1(posE) -> squaresum/1(E1)
  E/1 -> squaresum/3(E2)
  world/2(posN) -> squaresum/2(N1)
  Saturation/1 -> world/1(index)

== system IntegratedModel/Controller/Indexer/FindNearestIndex/ForwardSearch/Subsystem3 ==
  CurrentIndex : Inport
  E : Inport  Port=2
  N : Inport  Port=3
  Saturation : Saturate  UpperLimit=world.maxIndex  LowerLimit=1
  squaresum : Subsystem
  world : Subsystem
  Squsum : Outport
  wires:
  squaresum/1(squsum) -> Squsum/1
  CurrentIndex/1 -> Saturation/1
  N/1 -> squaresum/4(N2)
  world/1(posE) -> squaresum/1(E1)
  E/1 -> squaresum/3(E2)
  world/2(posN) -> squaresum/2(N1)
  Saturation/1 -> world/1(index)

== system IntegratedModel/Controller/Indexer/FindNearestIndex/ForwardSearch/Subsystem4 ==
  CurrentIndex : Inport
  E : Inport  Port=2
  N : Inport  Port=3
  Saturation : Saturate  UpperLimit=world.maxIndex  LowerLimit=1
  squaresum : Subsystem
  world : Subsystem
  Squsum : Outport
  wires:
  squaresum/1(squsum) -> Squsum/1
  CurrentIndex/1 -> Saturation/1
  N/1 -> squaresum/4(N2)
  world/1(posE) -> squaresum/1(E1)
  E/1 -> squaresum/3(E2)
  world/2(posN) -> squaresum/2(N1)
  Saturation/1 -> world/1(index)

== system IntegratedModel/Controller/Indexer/FindNearestIndex/ForwardSearch/Subsystem5 ==
  In1 : Inport
  In2 : Inport  Port=2
  Compare To Zero : simulink/Logic and Bit Operations/Compare To Zero  relop=<  OutDataTypeStr=boolean
  Minus : Sum  Inputs=+-
  In1isSmaller : Outport
  wires:
  In1/1 -> Minus/1
  In2/1 -> Minus/2
  Minus/1 -> Compare To Zero/1
  Compare To Zero/1 -> In1isSmaller/1

== system IntegratedModel/Controller/Indexer/FindNearestIndex/ForwardSearch/Subsystem6 ==
  In1 : Inport
  In2 : Inport  Port=2
  Compare To Zero : simulink/Logic and Bit Operations/Compare To Zero  relop=<  OutDataTypeStr=boolean
  Minus : Sum  Inputs=+-
  In1isSmaller : Outport
  wires:
  In1/1 -> Minus/1
  In2/1 -> Minus/2
  Minus/1 -> Compare To Zero/1
  Compare To Zero/1 -> In1isSmaller/1

== system IntegratedModel/Controller/Indexer/FindNearestIndex/ForwardSearch/Subsystem7 ==
  In1 : Inport
  In2 : Inport  Port=2
  Compare To Zero : simulink/Logic and Bit Operations/Compare To Zero  relop=<  OutDataTypeStr=boolean
  Minus : Sum  Inputs=+-
  In1isSmaller : Outport
  wires:
  In1/1 -> Minus/1
  In2/1 -> Minus/2
  Minus/1 -> Compare To Zero/1
  Compare To Zero/1 -> In1isSmaller/1

== system IntegratedModel/Controller/Indexer/FindNearestIndex/ForwardSearch/Subsystem8 ==
  In1 : Inport
  In2 : Inport  Port=2
  Compare To Zero : simulink/Logic and Bit Operations/Compare To Zero  relop=<  OutDataTypeStr=boolean
  Minus : Sum  Inputs=+-
  In1isSmaller : Outport
  wires:
  In1/1 -> Minus/1
  In2/1 -> Minus/2
  Minus/1 -> Compare To Zero/1
  Compare To Zero/1 -> In1isSmaller/1

== system IntegratedModel/Controller/Indexer/FindNearestIndex/ForwardSearch/Subsystem/squaresum ==
  E1 : Inport
  N1 : Inport  Port=2
  E2 : Inport  Port=3
  N2 : Inport  Port=4
  Minus : Sum  Inputs=+-
  Minus1 : Sum  Inputs=+-
  Plus : Sum
  Square : Math  Operator=square  SaturateOnIntegerOverflow=on
  Square1 : Math  Operator=square  SaturateOnIntegerOverflow=on
  squsum : Outport
  wires:
  N1/1 -> Minus1/1
  Minus/1 -> Square/1
  E1/1 -> Minus/1
  Plus/1 -> squsum/1
  Square1/1 -> Plus/2
  Minus1/1 -> Square1/1
  Square/1 -> Plus/1
  N2/1 -> Minus1/2
  E2/1 -> Minus/2

== system IntegratedModel/Controller/Indexer/FindNearestIndex/ForwardSearch/Subsystem/world ==
  index : Inport
  world.posE_m : Lookup_n-D  NumberOfTableDimensions=1  BreakpointsForDimension1=world.index  Table=world.posE_m  InternalRulePriority=Speed  RndMeth=Simplest  InputSameDT=on
  world.posN_m : Lookup_n-D  NumberOfTableDimensions=1  BreakpointsForDimension1=world.index  Table=world.posN_m  InternalRulePriority=Speed  RndMeth=Simplest  InputSameDT=on
  posE : Outport
  posN : Outport  Port=2
  wires:
  index/1 -> world.posN_m/1, world.posE_m/1
  world.posE_m/1 -> posE/1
  world.posN_m/1 -> posN/1

== system IntegratedModel/Controller/Indexer/FindNearestIndex/ForwardSearch/Subsystem1/squaresum ==
  E1 : Inport
  N1 : Inport  Port=2
  E2 : Inport  Port=3
  N2 : Inport  Port=4
  Minus : Sum  Inputs=+-
  Minus1 : Sum  Inputs=+-
  Plus : Sum
  Square : Math  Operator=square  SaturateOnIntegerOverflow=on
  Square1 : Math  Operator=square  SaturateOnIntegerOverflow=on
  squsum : Outport
  wires:
  N1/1 -> Minus1/1
  Minus/1 -> Square/1
  E1/1 -> Minus/1
  Plus/1 -> squsum/1
  Square1/1 -> Plus/2
  Minus1/1 -> Square1/1
  Square/1 -> Plus/1
  N2/1 -> Minus1/2
  E2/1 -> Minus/2

== system IntegratedModel/Controller/Indexer/FindNearestIndex/ForwardSearch/Subsystem1/world ==
  index : Inport
  world.posE_m : Lookup_n-D  NumberOfTableDimensions=1  BreakpointsForDimension1=world.index  Table=world.posE_m  InternalRulePriority=Speed  RndMeth=Simplest  InputSameDT=on
  world.posN_m : Lookup_n-D  NumberOfTableDimensions=1  BreakpointsForDimension1=world.index  Table=world.posN_m  InternalRulePriority=Speed  RndMeth=Simplest  InputSameDT=on
  posE : Outport
  posN : Outport  Port=2
  wires:
  index/1 -> world.posN_m/1, world.posE_m/1
  world.posE_m/1 -> posE/1
  world.posN_m/1 -> posN/1

== system IntegratedModel/Controller/Indexer/FindNearestIndex/ForwardSearch/Subsystem2/squaresum ==
  E1 : Inport
  N1 : Inport  Port=2
  E2 : Inport  Port=3
  N2 : Inport  Port=4
  Minus : Sum  Inputs=+-
  Minus1 : Sum  Inputs=+-
  Plus : Sum
  Square : Math  Operator=square  SaturateOnIntegerOverflow=on
  Square1 : Math  Operator=square  SaturateOnIntegerOverflow=on
  squsum : Outport
  wires:
  N1/1 -> Minus1/1
  Minus/1 -> Square/1
  E1/1 -> Minus/1
  Plus/1 -> squsum/1
  Square1/1 -> Plus/2
  Minus1/1 -> Square1/1
  Square/1 -> Plus/1
  N2/1 -> Minus1/2
  E2/1 -> Minus/2

== system IntegratedModel/Controller/Indexer/FindNearestIndex/ForwardSearch/Subsystem2/world ==
  index : Inport
  world.posE_m : Lookup_n-D  NumberOfTableDimensions=1  BreakpointsForDimension1=world.index  Table=world.posE_m  InternalRulePriority=Speed  RndMeth=Simplest  InputSameDT=on
  world.posN_m : Lookup_n-D  NumberOfTableDimensions=1  BreakpointsForDimension1=world.index  Table=world.posN_m  InternalRulePriority=Speed  RndMeth=Simplest  InputSameDT=on
  posE : Outport
  posN : Outport  Port=2
  wires:
  index/1 -> world.posN_m/1, world.posE_m/1
  world.posE_m/1 -> posE/1
  world.posN_m/1 -> posN/1

== system IntegratedModel/Controller/Indexer/FindNearestIndex/ForwardSearch/Subsystem3/squaresum ==
  E1 : Inport
  N1 : Inport  Port=2
  E2 : Inport  Port=3
  N2 : Inport  Port=4
  Minus : Sum  Inputs=+-
  Minus1 : Sum  Inputs=+-
  Plus : Sum
  Square : Math  Operator=square  SaturateOnIntegerOverflow=on
  Square1 : Math  Operator=square  SaturateOnIntegerOverflow=on
  squsum : Outport
  wires:
  N1/1 -> Minus1/1
  Minus/1 -> Square/1
  E1/1 -> Minus/1
  Plus/1 -> squsum/1
  Square1/1 -> Plus/2
  Minus1/1 -> Square1/1
  Square/1 -> Plus/1
  N2/1 -> Minus1/2
  E2/1 -> Minus/2

== system IntegratedModel/Controller/Indexer/FindNearestIndex/ForwardSearch/Subsystem3/world ==
  index : Inport
  world.posE_m : Lookup_n-D  NumberOfTableDimensions=1  BreakpointsForDimension1=world.index  Table=world.posE_m  InternalRulePriority=Speed  RndMeth=Simplest  InputSameDT=on
  world.posN_m : Lookup_n-D  NumberOfTableDimensions=1  BreakpointsForDimension1=world.index  Table=world.posN_m  InternalRulePriority=Speed  RndMeth=Simplest  InputSameDT=on
  posE : Outport
  posN : Outport  Port=2
  wires:
  index/1 -> world.posN_m/1, world.posE_m/1
  world.posE_m/1 -> posE/1
  world.posN_m/1 -> posN/1

== system IntegratedModel/Controller/Indexer/FindNearestIndex/ForwardSearch/Subsystem4/squaresum ==
  E1 : Inport
  N1 : Inport  Port=2
  E2 : Inport  Port=3
  N2 : Inport  Port=4
  Minus : Sum  Inputs=+-
  Minus1 : Sum  Inputs=+-
  Plus : Sum
  Square : Math  Operator=square  SaturateOnIntegerOverflow=on
  Square1 : Math  Operator=square  SaturateOnIntegerOverflow=on
  squsum : Outport
  wires:
  N1/1 -> Minus1/1
  Minus/1 -> Square/1
  E1/1 -> Minus/1
  Plus/1 -> squsum/1
  Square1/1 -> Plus/2
  Minus1/1 -> Square1/1
  Square/1 -> Plus/1
  N2/1 -> Minus1/2
  E2/1 -> Minus/2

== system IntegratedModel/Controller/Indexer/FindNearestIndex/ForwardSearch/Subsystem4/world ==
  index : Inport
  world.posE_m : Lookup_n-D  NumberOfTableDimensions=1  BreakpointsForDimension1=world.index  Table=world.posE_m  InternalRulePriority=Speed  RndMeth=Simplest  InputSameDT=on
  world.posN_m : Lookup_n-D  NumberOfTableDimensions=1  BreakpointsForDimension1=world.index  Table=world.posN_m  InternalRulePriority=Speed  RndMeth=Simplest  InputSameDT=on
  posE : Outport
  posN : Outport  Port=2
  wires:
  index/1 -> world.posN_m/1, world.posE_m/1
  world.posE_m/1 -> posE/1
  world.posN_m/1 -> posN/1
